simulink model "hardwareControl"  (R2021b)
settings: Solver=FixedStepAuto  StartTime=0.0  StopTime=inf  RelTol=1e-3  EnableMultiTasking=on
PostLoadFcn:
  | run("modelParameters.m")
values from neighbouring files (symbols this model uses):
  Ts = 0.01    [modelParameters.m]
libraries: arduinomotorcarrierlib x3, simulink x1, eeGeneralControl x1, arduinosensorlib x1, mkrmotorcarrierlib x1
settings Model: ExtModeTrigDuration=2  Creator=bkhusain  LastModifiedBy=adoor_
settings SolverCC: AlgebraicLoopSolver=TrustRegion
settings OptimizationCC: EnhancedBackFolding=on  PassReuseOutputArgsThreshold=0  MaxStackSize=64  OptimizeBlockOrder=speed  DifferentSizesBufferReuse=on  OptimizationCustomize=off
settings DebuggingCC: ParameterTunabilityLossMsg=error  SFMachineParentedDataDiag=warning
settings HardwareCC: ProdBitPerPointer=32  ProdBitPerSizeT=32  ProdBitPerPtrDiffT=32  ProdLargestAtomicInteger=Long  ProdLargestAtomicFloat=Double  ProdWordSize=32  ProdHWDeviceType=ARM Compatible->ARM Cortex  UseEmbeddedCoderFeatures=off  UseSimulinkCoderFeatures=off
settings SFSimCC: MATLABDynamicMemAlloc=off
settings RTWCC: Description=Embedded Coder  SystemTargetFile=ert.tlc  HardwareBoard=Arduino Nano 33 IoT  TemplateMakefile=ert_default_tmf  Toolchain=Arduino ARM  BuildConfiguration=Faster Runs
settings CodeAppCC: ForceParamTrailComments=on  OperatorAnnotations=on
settings ERTTargetCC: ERTCustomFileBanners=off  SupportContinuousTime=on  SupportNonInlinedSFcns=on  RemoveResetFunc=off  SupportVariableSizeSignals=on  ModelStepFunctionPrototypeControlCompliant=off  ExtModeStaticAllocSize=8192

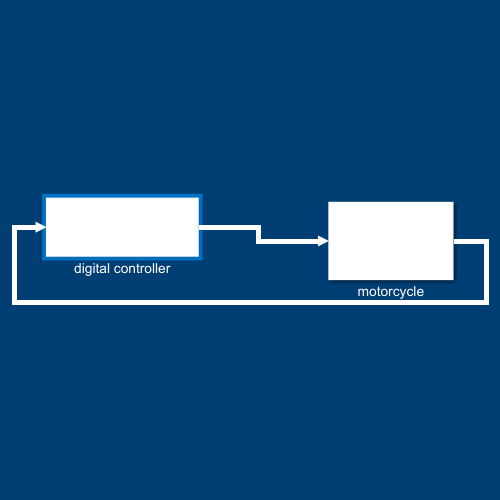
[thumbnail: Simulink's stored preview of the top-level diagram]
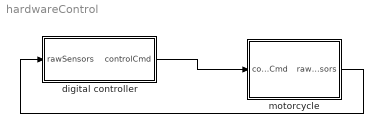
== system hardwareControl ==
  digital controller : Subsystem
      mask Display: image('$imagefile'); % Use "Edit Image" on toolstrip to change.
  motorcycle : Subsystem
      mask Display: image('$imagefile'); % Use "Edit Image" on toolstrip to change.
  wires:
  digital controller/1(controlCmd) -> motorcycle/1(controlCmd)
  motorcycle/1(rawSensors) -> digital controller/1(rawSensors)

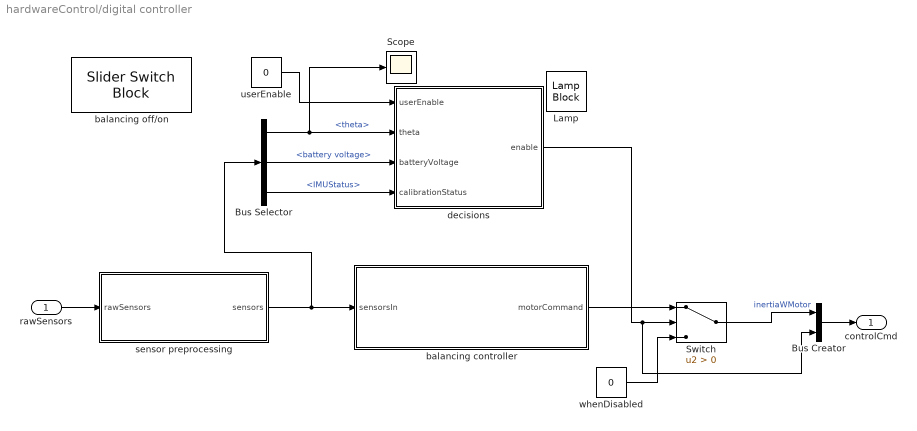
== system hardwareControl/digital controller ==
  rawSensors : Inport
  Bus Creator : BusCreator  Inputs=2
  Bus Selector : BusSelector  OutputSignals=theta,battery voltage,IMUStatus
  Lamp : LampBlock
  Scope : Scope
  Switch : Switch  Criteria=u2 > Threshold
  balancing controller : Subsystem
  balancing off/on : SliderSwitchBlock  LabelPosition=Hide
      settings: Values={{'Off', 'On'}, [0 1]}
  decisions : Stateflow chart  TreatAsAtomicUnit=on
  sensor preprocessing : Subsystem
  userEnable : Constant  Value=0  SampleTime=Ts
  whenDisabled : Constant  Value=0  SampleTime=Ts
  controlCmd : Outport
  wires:
  Switch/1 -> Bus Creator/1  "inertiaWMotor"
  Bus Creator/1 -> controlCmd/1
  rawSensors/1 -> sensor preprocessing/1(rawSensors)
  sensor preprocessing/1(sensors) -> balancing controller/1(sensorsIn), Bus Selector/1
  whenDisabled/1 -> Switch/3
  decisions/1(enable) -> Switch/2, Bus Creator/2
  Bus Selector/1 -> Scope/1, decisions/2(theta)  "<theta>"
  Bus Selector/2 -> decisions/3(batteryVoltage)  "<battery voltage>"
  Bus Selector/3 -> decisions/4(calibrationStatus)  "<IMUStatus>"
  userEnable/1 -> decisions/1(userEnable)
  balancing controller/1(motorCommand) -> Switch/1

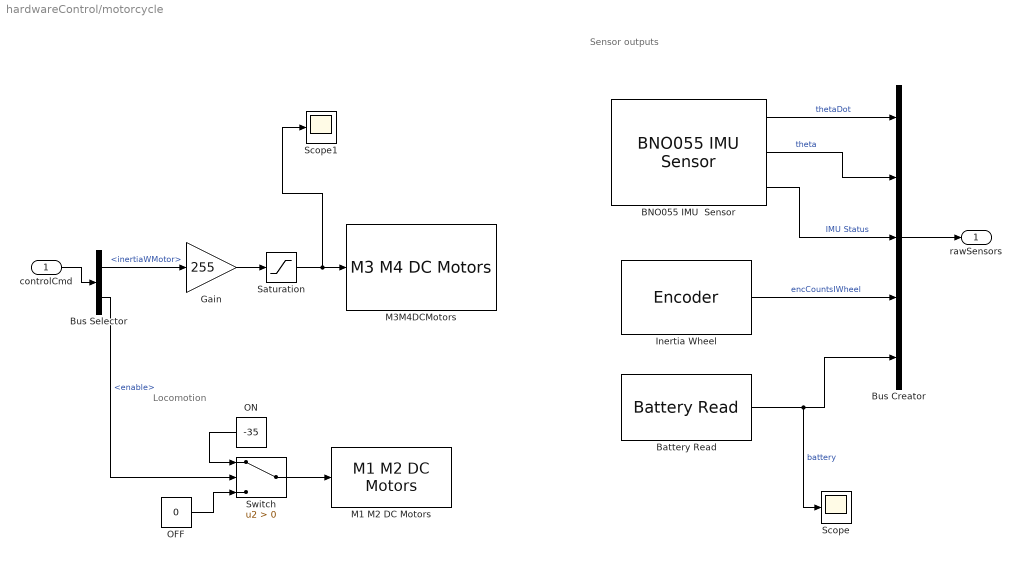
== system hardwareControl/motorcycle ==
  note: Locomotion
  note: Sensor outputs
  controlCmd : Inport
  BNO055 IMU  Sensor : arduinosensorlib/BNO055 IMU Sensor  SlaveAddress=0x28  OperationMode=Fusion  Accel=off  AngularRate=on  MagField=off  EulerAngles=on  Quat=off  LinearAccel=off  GravityVector=off  Status=on  AccelRange=4G  AccelBW=62.5 Hz  GyroRange=2000 dps  GyroBW=32 Hz  MagODR=10 Hz  SampleTime=Ts  blockPlatform=ARDUINO
      settings: SourceProductName=Simulink Support for Arduino Sensors
  Battery Read : arduinomotorcarrierlib/Battery Read  SlaveAddress=uint8( hex2dec( '66' ) )  blockPlatform=ARDUINO  SampleTime=Ts
      settings: SourceProductBaseCode=ARDUINO
  Bus Creator : BusCreator  Inputs=5
  Bus Selector : BusSelector  OutputSignals=inertiaWMotor,enable
  Gain : Gain  Gain=255
  Inertia Wheel : arduinomotorcarrierlib/Encoder  SlaveAddress=uint8( hex2dec( '66' ) )  blockPlatform=ARDUINO  Encoder=1  ShowSpeed=off  ResetOption=on  SampleTime=Ts
      settings: SourceProductName=Simulink Support for Arduino MKR Motor Carrier
  M1 M2 DC Motors : arduinomotorcarrierlib/M1 M2 DC Motors  SlaveAddress=uint8( hex2dec( '66' ) )  blockPlatform=ARDUINO  MotorNumber=M2  MotorCarrierPWMFreq=100
      settings: SourceProductBaseCode=ARDUINO
  M3M4DCMotors : mkrmotorcarrierlib/M3 M4 DC Motors  MotorNumber=M3  forwardPinNumber=3  reversePinNumber=2
      settings: SourceProductName=Simulink Support for Arduino MKR Motor Carrier
  OFF : Constant  Value=0
  ON : Constant  Value=-35
  Saturation : Saturate  UpperLimit=255  LowerLimit=-255
  Scope : Scope
  Scope1 : Scope
  Switch : Switch  Criteria=u2 > Threshold
  rawSensors : Outport
  wires:
  BNO055 IMU  Sensor/1 -> Bus Creator/1  "thetaDot"
  BNO055 IMU  Sensor/2 -> Bus Creator/2  "theta"
  BNO055 IMU  Sensor/3 -> Bus Creator/3  "IMU Status"
  Inertia Wheel/1 -> Bus Creator/4  "encCountsIWheel"
  Battery Read/1 -> Scope/1, Bus Creator/5  "battery"
  Bus Creator/1 -> rawSensors/1
  controlCmd/1 -> Bus Selector/1
  Gain/1 -> Saturation/1
  Bus Selector/1 -> Gain/1  "<inertiaWMotor>"
  Saturation/1 -> Scope1/1, M3M4DCMotors/1
  ON/1 -> Switch/1
  OFF/1 -> Switch/3
  Switch/1 -> M1 M2 DC Motors/1
  Bus Selector/2 -> Switch/2  "<enable>"

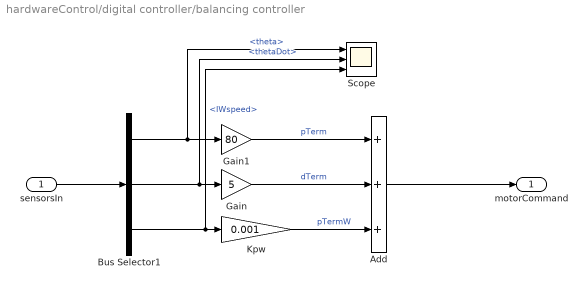
== system hardwareControl/digital controller/balancing controller ==
  sensorsIn : Inport
  Add : Sum  Inputs=+++
  Bus Selector1 : BusSelector  OutputSignals=theta,thetaDot,IWspeed
  Gain : Gain  Gain=5
  Gain1 : Gain  Gain=80
  Kpw : Gain  Gain=0.001
  Scope : Scope  NumInputPorts=3
  motorCommand : Outport
  wires:
  Bus Selector1/3 -> Scope/3, Kpw/1  "<IWspeed>"
  Kpw/1 -> Add/3  "pTermW"
  Gain/1 -> Add/2  "dTerm"
  Bus Selector1/2 -> Scope/2, Gain/1  "<thetaDot>"
  Bus Selector1/1 -> Scope/1, Gain1/1  "<theta>"
  sensorsIn/1 -> Bus Selector1/1
  Add/1 -> motorCommand/1
  Gain1/1 -> Add/1  "pTerm"

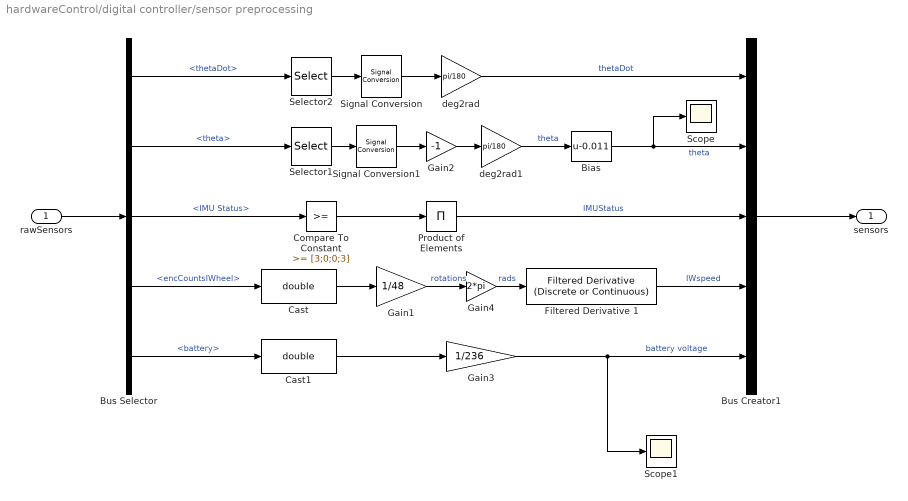
== system hardwareControl/digital controller/sensor preprocessing ==
  rawSensors : Inport
  Bias : Bias  Bias=-0.011
  Bus Creator1 : BusCreator  Inputs=5
  Bus Selector : BusSelector  OutputSignals=thetaDot,theta,IMU Status,encCountsIWheel,battery
  Cast : DataTypeConversion  OutDataTypeStr=double
  Cast1 : DataTypeConversion  OutDataTypeStr=double
  Compare To Constant : simulink/Logic and Bit Operations/Compare To Constant  relop=>=  const=[3;0;0;3]  OutDataTypeStr=boolean
  Filtered Derivative 1 : eeGeneralControl/Filtered Derivative (Discrete or Continuous)  K=1  T=0.1  B=inf  A=-inf  minRatio=10  init_option=Inherited from block input  x0=0  Ts=Ts
      settings: SourceProductBaseCode=PS
  Gain1 : Gain  Gain=1/48
  Gain2 : Gain  Gain=-1
  Gain3 : Gain  Gain=1/236
  Gain4 : Gain  Gain=2*pi
  Product of Elements : Product  Inputs=*
  Scope : Scope
  Scope1 : Scope
  Selector1 : Selector  InputPortWidth=3  IndexOptions=Index vector (dialog)  Indices=[2]  OutputSizes=1
  Selector2 : Selector  InputPortWidth=3  IndexOptions=Index vector (dialog)  Indices=[2]  OutputSizes=1
  Signal Conversion : SignalConversion  OverrideOpt=off
  Signal Conversion1 : SignalConversion  OverrideOpt=off
  deg2rad : Gain  Gain=pi/180
  deg2rad1 : Gain  Gain=pi/180
  sensors : Outport
  wires:
  Bus Selector/4 -> Cast/1  "<encCountsIWheel>"
  Compare To Constant/1 -> Product of Elements/1
  Bus Selector/5 -> Cast1/1  "<battery>"
  Selector2/1 -> Signal Conversion/1
  Bus Selector/2 -> Selector1/1  "<theta>"
  Selector1/1 -> Signal Conversion1/1
  Cast1/1 -> Gain3/1
  Bus Selector/3 -> Compare To Constant/1  "<IMU Status>"
  rawSensors/1 -> Bus Selector/1
  Product of Elements/1 -> Bus Creator1/3  "IMUStatus"
  Filtered Derivative 1/1 -> Bus Creator1/4  "IWspeed"
  deg2rad1/1 -> Bias/1  "theta"
  Bus Selector/1 -> Selector2/1  "<thetaDot>"
  Gain3/1 -> Scope1/1, Bus Creator1/5  "battery voltage"
  Bus Creator1/1 -> sensors/1
  Signal Conversion1/1 -> Gain2/1
  Gain2/1 -> deg2rad1/1
  Signal Conversion/1 -> deg2rad/1
  Cast/1 -> Gain1/1
  Gain1/1 -> Gain4/1  "rotations"
  Gain4/1 -> Filtered Derivative 1/1  "rads"
  deg2rad/1 -> Bus Creator1/1  "thetaDot"
  Bias/1 -> Scope/1, Bus Creator1/2  "theta"

== stateflow chart hardwareControl/digital controller/decisions ==
  state checkIMUCalib [parallel]
    settings: executionOrder=2
    state imuNotCalibrated
      entry:
      IMUCalibrated = false;
    state imuCalibrated
      entry:
      IMUCalibrated = true;
    (default) -> imuNotCalibrated
    imuNotCalibrated -> imuCalibrated : [calibrationStatus == true]
  state checkFallen [parallel]
    settings: executionOrder=1
    state fallen
      entry: upright = false
    state standing
      entry: upright = true
    (default) -> fallen
    fallen -> standing : [abs(theta) < 0.25]
    standing -> fallen : [abs(theta) > 0.25]
  state checkBattery [parallel]
    settings: executionOrder=3
    state batteryNotCharged
      entry:
      batteryOK = false;
    state batteryCharged
      entry:
      batteryOK = true;
    (default) -> batteryNotCharged
    batteryCharged -> batteryNotCharged : [batteryVoltage < 3.0]
    batteryNotCharged -> batteryCharged : [batteryVoltage >= 3.0]
  state calculateEnable [parallel]
    settings: executionOrder=4
    state disableControl
      entry: enable = false
    state enableControl
      entry: enable = true
    (default) -> disableControl
    disableControl -> enableControl : [userEnable&& batteryOK && IMUCalibrated && upright]
    enableControl -> disableControl : [not(userEnable) || not(batteryOK) || not(IMUCalibrated) || not(upright)]
  data: userEnable input; theta input; enable output; batteryVoltage input; calibrationStatus input; upright local; IMUCalibrated local; batteryOK local
